simulink model "LinearRLC1DiscreteModel"  (R2014a)
settings: Solver=FixedStepDiscrete  StartTime=0.0  StopTime=5  FixedStep=0.1  RelTol=1e-3
settings Model: Creator=SH343  LastModifiedBy=SH343
settings DataIOCC: SignalLoggingSaveFormat=ModelDataLogs
settings DebuggingCC: MultiTaskDSMMsg=warning  MultiTaskCondExecSysMsg=none
settings RTWCC: IncludeERTFirstTime=on

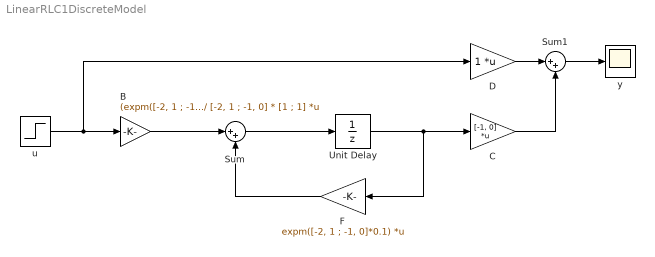
== system LinearRLC1DiscreteModel ==
  B : Gain  Gain=(expm([-2, 1 ; -1, 0] * 0.1) - eye(2)) / [-2, 1 ; -1, 0] * [1 ; 1]  Multiplication=Matrix(K*u)
  C : Gain  Gain=[-1, 0]  Multiplication=Matrix(K*u)
  D : Gain  Multiplication=Matrix(K*u)
  F : Gain  Gain=expm([-2, 1 ; -1, 0]*0.1)  Multiplication=Matrix(K*u)
  Sum : Sum  Inputs=|++
  Sum1 : Sum  Inputs=|++
  Unit Delay : UnitDelay  SampleTime=-1
  u : Step  Time=0  SampleTime=0
  y : Scope
  wires:
  u/1 -> D/1, B/1
  Unit Delay/1 -> F/1, C/1
  Sum/1 -> Unit Delay/1
  F/1 -> Sum/2
  B/1 -> Sum/1
  C/1 -> Sum1/2
  Sum1/1 -> y/1
  D/1 -> Sum1/1
